simulink model "full_car_ride"  (R2026a)
settings: Solver=VariableStepAuto  StopTime=10
settings Model: Creator=ANDALIBM  LastModifiedBy=eonra
settings DebuggingCC: SignalResolutionControl=TryResolveAllWithWarning
settings SimscapeCC: SimscapeNominalValues="[{\"value\":\"1\",\"unit\":\"A\"},{\"value\":\"1\",\"unit\":\"bar\"},{\"value\":\"1\",\"unit\":\"cm^2\"},{\"value\":\"1\",\"unit\":\"cm^3/s\"},{\"value\":\"1\",\"unit\":\"kJ/kg\"},{\"value\":\"1\",\"unit\":\"kW\"},{\"value\":\"1\",\"unit\":\"l\"},{\"value\":\"1\",\"unit\":\"N\"},{\"value\":\"1\",\"unit\":\"N*m\"},{\"value\":\"1\",\"unit\":\"V\"}]"  SimscapeLogType=none  SimscapeLogDataHistory=5000  SimscapeLogDecimation=1

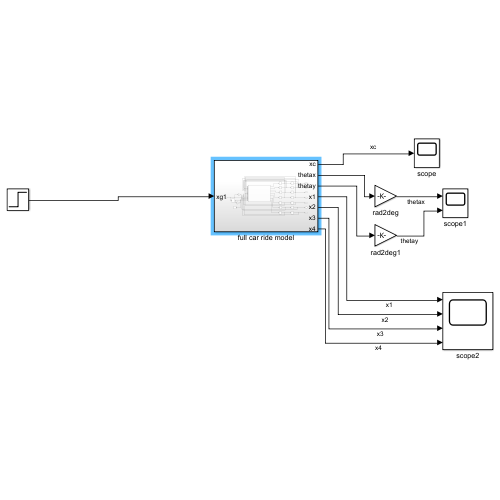
[thumbnail: Simulink's stored preview of the top-level diagram]
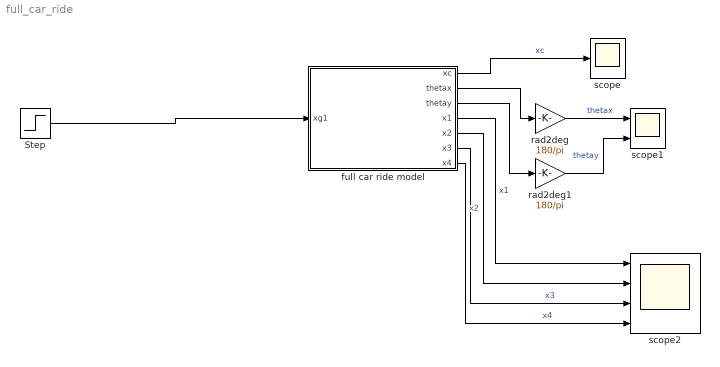
== system full_car_ride ==
  Step : Step  Time=0  FinalValue=0.05  SampleTime=0
  full car ride model : Subsystem
  rad2deg : Gain  Gain=180/pi
  rad2deg1 : Gain  Gain=180/pi
  scope : Scope
      settings: SampleTime=0.01  ActiveDisplayYMinimum=-0.0039742831658568685  ActiveDisplayYMaximum=0.035768548492711827  DataLoggingVariableName=xc  DataLoggingSaveFormat=Array
  scope1 : Scope  NumInputPorts=2
      settings: SampleTime=0.01  ActiveDisplayYMinimum=-3.6024468981656761  ActiveDisplayYMaximum=0.49696645999718525  DataLoggingSaveFormat=Structure
  scope2 : Scope  NumInputPorts=4
      settings: SampleTime=0.01  ActiveDisplayYMinimum=-0.013141613362289015  ActiveDisplayYMaximum=0.065688476863264844  DataLoggingVariableName=ScopeData2  DataLoggingSaveFormat=Structure
  wires:
  full car ride model/1(xc) -> scope/1  "xc"
  full car ride model/2(thetax) -> rad2deg/1
  rad2deg/1 -> scope1/1  "thetax"
  full car ride model/3(thetay) -> rad2deg1/1
  rad2deg1/1 -> scope1/2  "thetay"
  full car ride model/4(x1) -> scope2/1  "x1"
  full car ride model/7(x4) -> scope2/4  "x4"
  full car ride model/6(x3) -> scope2/3  "x3"
  full car ride model/5(x2) -> scope2/2  "x2"
  Step/1 -> full car ride model/1(xg1)

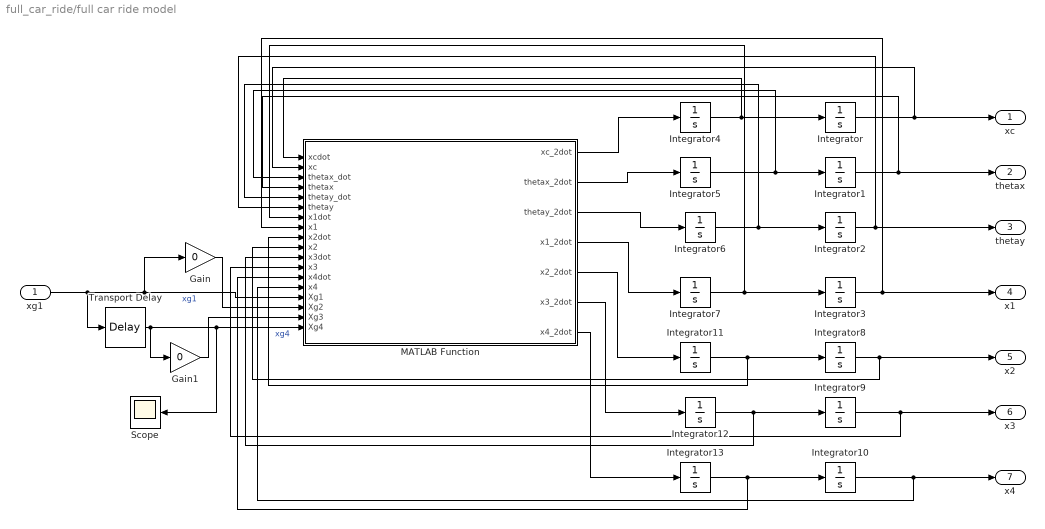
== system full_car_ride/full car ride model ==
  xg1 : Inport
  Gain : Gain  Gain=0
  Gain1 : Gain  Gain=0
  Integrator{,1..13} (14 alike) : Integrator
  MATLAB Function : MATLAB Function  TreatAsAtomicUnit=on
  Scope : Scope
      settings: ActiveDisplayYMinimum=-0.0089  ActiveDisplayYMaximum=0.28771  DataLoggingVariableName=ScopeData3
  Transport Delay : TransportDelay  DelayTime=1.6/15
  xc : Outport
  thetax : Outport  Port=2
  thetay : Outport  Port=3
  x1 : Outport  Port=4
  x2 : Outport  Port=5
  x3 : Outport  Port=6
  x4 : Outport  Port=7
  wires:
  Integrator/1 -> MATLAB Function/2(xc), xc/1
  Integrator1/1 -> MATLAB Function/4(thetax), thetax/1
  Integrator2/1 -> MATLAB Function/6(thetay), thetay/1
  Integrator3/1 -> MATLAB Function/8(x1), x1/1
  Integrator7/1 -> MATLAB Function/7(x1dot), Integrator3/1
  Integrator6/1 -> MATLAB Function/5(thetay_dot), Integrator2/1
  Integrator5/1 -> MATLAB Function/3(thetax_dot), Integrator1/1
  Integrator4/1 -> MATLAB Function/1(xcdot), Integrator/1
  xg1/1 -> Gain/1, MATLAB Function/15(Xg1), Transport Delay/1  "xg1"
  Transport Delay/1 -> Gain1/1, MATLAB Function/18(Xg4), Scope/1  "xg4"
  Integrator11/1 -> MATLAB Function/9(x2dot), Integrator8/1
  Integrator12/1 -> MATLAB Function/11(x3dot), Integrator9/1
  Integrator13/1 -> MATLAB Function/13(x4dot), Integrator10/1
  Integrator10/1 -> MATLAB Function/14(x4), x4/1
  Integrator9/1 -> MATLAB Function/12(x3), x3/1
  Integrator8/1 -> MATLAB Function/10(x2), x2/1
  MATLAB Function/1(xc_2dot) -> Integrator4/1
  MATLAB Function/2(thetax_2dot) -> Integrator5/1
  MATLAB Function/3(thetay_2dot) -> Integrator6/1
  MATLAB Function/4(x1_2dot) -> Integrator7/1
  MATLAB Function/5(x2_2dot) -> Integrator11/1
  MATLAB Function/6(x3_2dot) -> Integrator12/1
  MATLAB Function/7(x4_2dot) -> Integrator13/1
  Gain/1 -> MATLAB Function/16(Xg2)
  Gain1/1 -> MATLAB Function/17(Xg3)

== matlab function full_car_ride/full car ride model/MATLAB Function ==
  settings: sampleTime=1
  data: xcdot input; xc input; thetax_dot input; thetax input; thetay_dot input; thetay input; x1dot input; xc_2dot output; x1 input; thetax_2dot output; thetay_2dot output; x1_2dot output; x2_2dot output; x2dot input; x2 input; x3dot input; x3 input; x4dot input; x4 input; Xg1 input; Xg2 input; Xg3 input; Xg4 input; x3_2dot output; x4_2dot output
function [xc_2dot, thetax_2dot, thetay_2dot, x1_2dot, x2_2dot, x3_2dot, x4_2dot] = fcn(...
    xcdot, xc, thetax_dot, thetax, thetay_dot, thetay, ...
    x1dot, x1, x2dot, x2, x3dot, x3, x4dot, x4, ...
    Xg1, Xg2, Xg3, Xg4)


a=0.88;
b=0.72;
c=0.6;
d=0.6;
M=250;
Ixx= 58;
Iyy= 190;
m1= 12.5;
m2= 12.5;
m3= 12.5;
m4= 12.5;
K1= 18034.39 ;
K2= 18034.39 ;
K3= 16216.42;
K4= 16216.42;
C1= 1501.12 ;
C2= 1501.12 ;
C3= 3620.33;
C4= 3620.33;
Kt1= 197321.95;
Kt2=  197321.95 ;
Kt3=   180049.32 ;
Kt4=   180049.32;


xc_2dot = ( K1*(x1 - (xc - a*thetay - c*thetax)) + C1*(x1dot - (xcdot - a*thetay_dot - c*thetax_dot)) + ...
            K2*(x2 - (xc - a*thetay + d*thetax)) + C2*(x2dot - (xcdot - a*thetay_dot + d*thetax_dot)) + ...
            K3*(x3 - (xc + b*thetay + d*thetax)) + C3*(x3dot - (xcdot + b*thetay_dot + d*thetax_dot)) + ...
            K4*(x4 - (xc + b*thetay - c*thetax)) + C4*(x4dot - (xcdot + b*thetay_dot - c*thetax_dot)) ) / M;

thetax_2dot = ( d * ( K2*(x2 - (xc - a*thetay + d*thetax)) + C2*(x2dot - (xcdot - a*thetay_dot + d*thetax_dot)) + ...
                      K3*(x3 - (xc + b*thetay + d*thetax)) + C3*(x3dot - (xcdot + b*thetay_dot + d*thetax_dot)) ) - ...
                c * ( K1*(x1 - (xc - a*thetay - c*thetax)) + C1*(x1dot - (xcdot - a*thetay_dot - c*thetax_dot)) + ...
                      K4*(x4 - (xc + b*thetay - c*thetax)) + C4*(x4dot - (xcdot + b*thetay_dot - c*thetax_dot)) ) ) / Ixx;

thetay_2dot = ( b * ( K3*(x3 - (xc + b*thetay + d*thetax)) + C3*(x3dot - (xcdot + b*thetay_dot + d*thetax_dot)) + ...
                      K4*(x4 - (xc + b*thetay - c*thetax)) + C4*(x4dot - (xcdot + b*thetay_dot - c*thetax_dot)) ) - ...
                a * ( K1*(x1 - (xc - a*thetay - c*thetax)) + C1*(x1dot - (xcdot - a*thetay_dot - c*thetax_dot)) + ...
                      K2*(x2 - (xc - a*thetay + d*thetax)) + C2*(x2dot - (xcdot - a*thetay_dot + d*thetax_dot)) ) ) / Iyy;

x1_2dot = ( -K1*(x1 - (xc - a*thetay - c*thetax)) - C1*(x1dot - (xcdot - a*thetay_dot - c*thetax_dot)) + Kt1*(Xg1 - x1) ) / m1;
x2_2dot = ( -K2*(x2 - (xc - a*thetay + d*thetax)) - C2*(x2dot - (xcdot - a*thetay_dot + d*thetax_dot)) + Kt2*(Xg2 - x2) ) / m2;
x3_2dot = ( -K3*(x3 - (xc + b*thetay + d*thetax)) - C3*(x3dot - (xcdot + b*thetay_dot + d*thetax_dot)) + Kt3*(Xg3 - x3) ) / m3;
x4_2dot = ( -K4*(x4 - (xc + b*thetay - c*thetax)) - C4*(x4dot - (xcdot + b*thetay_dot - c*thetax_dot)) + Kt4*(Xg4 - x4) ) / m4;


end
